simulink model "ADAS_Main"  (R2024b)
settings: Solver=ode4  StartTime=0.01  StopTime=20.0  RelTol=1e-3
libraries: simulink x2, SignalEditorBlockLib x1
settings Model: Creator=us  LastModifiedBy=us
settings DataIOCC: ReturnWorkspaceOutputs=off

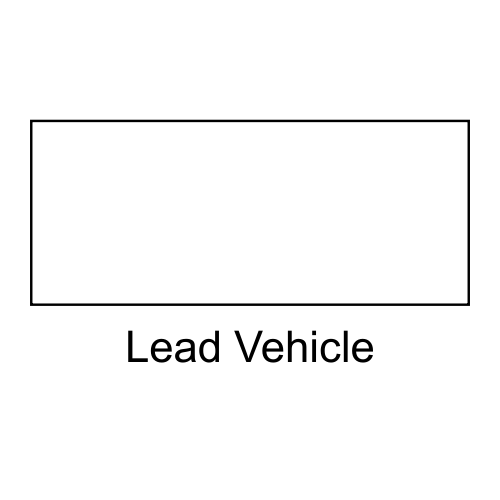
[thumbnail: Simulink's stored preview of the top-level diagram]
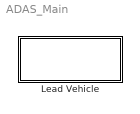
== system ADAS_Main ==
  Lead Vehicle : Subsystem

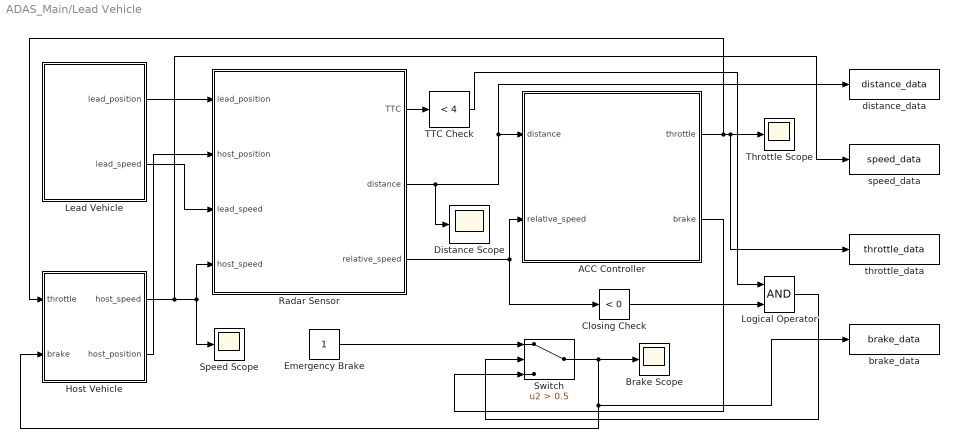
== system ADAS_Main/Lead Vehicle ==
  ACC Controller : Subsystem
  Brake Scope : Scope
  Closing Check : simulink/Logic and Bit Operations/Compare To Constant  relop=<  const=0  OutDataTypeStr=boolean
  Distance Scope : Scope
  Emergency Brake : Constant
  Host Vehicle : Subsystem
  Lead Vehicle : Subsystem
  Logical Operator : Logic  AllPortsSameDT=off  OutDataTypeStr=boolean
  Radar Sensor : Subsystem
  Speed Scope : Scope
  Switch : Switch  Criteria=u2 > Threshold  Threshold=0.5  SaturateOnIntegerOverflow=off  InputSameDT=off
  TTC Check : simulink/Logic and Bit Operations/Compare To Constant  relop=<  const=4  OutDataTypeStr=boolean
  Throttle Scope : Scope
  brake_data : ToWorkspace  VariableName=brake_data  SaveFormat=Structure With Time  SampleTime=-1
  distance_data : ToWorkspace  VariableName=distance_data  SaveFormat=Structure With Time  SampleTime=-1
  speed_data : ToWorkspace  VariableName=speed_data  SaveFormat=Structure With Time  SampleTime=-1
  throttle_data : ToWorkspace  VariableName=throttle_data  SaveFormat=Structure With Time  SampleTime=-1
  wires:
  Host Vehicle/1(host_speed) -> speed_data/1, Speed Scope/1, Radar Sensor/4(host_speed)
  Host Vehicle/2(host_position) -> Radar Sensor/2(host_position)
  Lead Vehicle/1(lead_position) -> Radar Sensor/1(lead_position)
  Lead Vehicle/2(lead_speed) -> Radar Sensor/3(lead_speed)
  ACC Controller/1("throttle ") -> Throttle Scope/1, throttle_data/1, Host Vehicle/1(throttle)
  ACC Controller/2(brake) -> Switch/3
  Radar Sensor/2(distance) -> ACC Controller/1(distance), distance_data/1, Distance Scope/1
  Radar Sensor/3(relative_speed) -> Closing Check/1, ACC Controller/2(relative_speed)
  Radar Sensor/1(TTC) -> TTC Check/1
  TTC Check/1 -> Logical Operator/1
  Emergency Brake/1 -> Switch/1
  Switch/1 -> brake_data/1, Host Vehicle/2(brake), Brake Scope/1
  Closing Check/1 -> Logical Operator/2
  Logical Operator/1 -> Switch/2

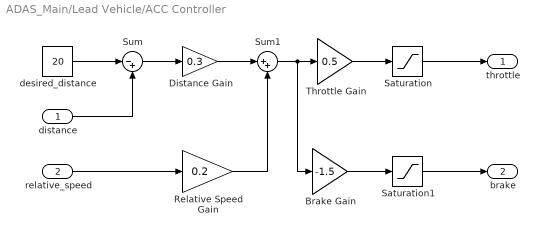
== system ADAS_Main/Lead Vehicle/ACC Controller ==
  distance : Inport
  relative_speed : Inport  Port=2
  Brake Gain : Gain  Gain=-1.5
  Distance Gain : Gain  Gain=0.3
  Relative Speed Gain : Gain  Gain=0.2
  Saturation : Saturate  UpperLimit=1  LowerLimit=0
  Saturation1 : Saturate  UpperLimit=1  LowerLimit=0
  Sum : Sum  Inputs=|-+
  Sum1 : Sum  Inputs=|++
  Throttle Gain : Gain  Gain=0.5
  desired_distance : Constant  Value=20
  "throttle " : Outport
  brake : Outport  Port=2
  wires:
  desired_distance/1 -> Sum/1
  distance/1 -> Sum/2
  Brake Gain/1 -> Saturation1/1
  Saturation1/1 -> brake/1
  Saturation/1 -> "throttle "/1
  relative_speed/1 -> Relative Speed Gain/1
  Relative Speed Gain/1 -> Sum1/2
  Sum1/1 -> Brake Gain/1, Throttle Gain/1
  Sum/1 -> Distance Gain/1
  Distance Gain/1 -> Sum1/1
  Throttle Gain/1 -> Saturation/1

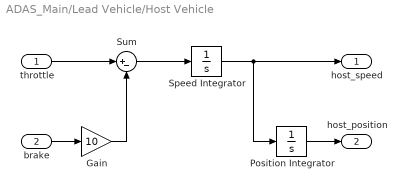
== system ADAS_Main/Lead Vehicle/Host Vehicle ==
  throttle : Inport
  brake : Inport  Port=2
  Gain : Gain  Gain=10
  Position Integrator : Integrator
  Speed Integrator : Integrator  InitialCondition=15
  Sum : Sum  Inputs=|+-
  host_speed : Outport
  host_position : Outport  Port=2
  wires:
  throttle/1 -> Sum/1
  Sum/1 -> Speed Integrator/1
  Speed Integrator/1 -> host_speed/1, Position Integrator/1
  Position Integrator/1 -> host_position/1
  Gain/1 -> Sum/2
  brake/1 -> Gain/1

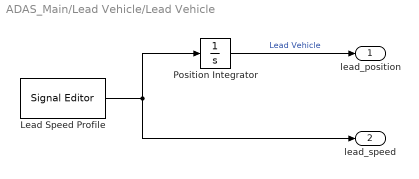
== system ADAS_Main/Lead Vehicle/Lead Vehicle ==
  Lead Speed Profile : SignalEditorBlockLib/Signal Editor  FileName=C:\Users\us\Desktop\Projects\ADAS_MATLAB_Project\resources\lead_speed_profile.mat  ActiveScenario=Scenario  ActiveSignal=Signal 1  IsBus=off  OutputBusObjectStr=Bus: BusObject  SampleTime=0  Interpolate=off  ZeroCross=off  OutputAfterFinalValue=Setting to zero  Unit=inherit  PreserveSignalName=on  ApplySigPropsToAllScenarios=on  ApplySigPropsToAllSignals=off
  Position Integrator : Integrator
  lead_position : Outport
  lead_speed : Outport  Port=2
  wires:
  Position Integrator/1 -> lead_position/1  "Lead Vehicle"
  Lead Speed Profile/1 -> lead_speed/1, Position Integrator/1

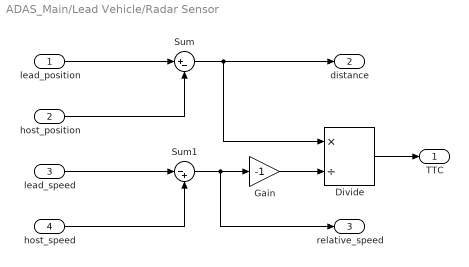
== system ADAS_Main/Lead Vehicle/Radar Sensor ==
  lead_position : Inport
  host_position : Inport  Port=2
  lead_speed : Inport  Port=3
  host_speed : Inport  Port=4
  Divide : Product  Inputs=*/
  Gain : Gain  Gain=-1
  Sum : Sum  Inputs=|+-
  Sum1 : Sum  Inputs=|-+
  TTC : Outport
  distance : Outport  Port=2
  relative_speed : Outport  Port=3
  wires:
  lead_position/1 -> Sum/1
  host_position/1 -> Sum/2
  Sum/1 -> distance/1, Divide/1
  lead_speed/1 -> Sum1/1
  host_speed/1 -> Sum1/2
  Sum1/1 -> Gain/1, relative_speed/1
  Divide/1 -> TTC/1
  Gain/1 -> Divide/2
